simulink model "simu_MA_lev"  (R2020a)
settings: Solver=VariableStepAuto  StartTime=0.0  StopTime=1972  RelTol=1e-3
values from neighbouring files (symbols this model uses):
  planta = tftp1    [ensMA_pontoOperacao_Limite.m]    (also in lev2.m = tftp5)
  t_rp = showRegPerm(init(1:end), vecTP13, vecIter, vecIR, 'TP13')    [ensMA_levModelo_TxI_noMaisLinear.m]    (also in ensMA_pontoOperacao_Limite.m = showRegPerm(init(1:end), vecTP1,vecIter, vecIR, 'TP1'); lev2.m = showRegPerm(init(1:end), vecTP5,vecIter, vecIR, 'TP5'))
settings Model: Creator=jricl  LastModifiedBy=User
settings DebuggingCC: SFMachineParentedDataDiag=error

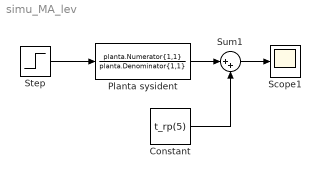
== system simu_MA_lev ==
  Constant : Constant  Value=t_rp(5)
  Planta sysident : TransferFcn  Numerator=planta.Numerator{1,1}  Denominator=planta.Denominator{1,1}
  Scope1 : Scope
  Step : Step  Time=0  After=0.044  SampleTime=1
  Sum1 : Sum  Inputs=|++
  wires:
  Constant/1 -> Sum1/2
  Sum1/1 -> Scope1/1
  Planta sysident/1 -> Sum1/1
  Step/1 -> Planta sysident/1
